simulink model "Simulation"  (R2014b)
settings: Solver=ode3  SolverMode=SingleTasking  StartTime=0.0  StopTime=Sim_time  FixedStep=0.02  RelTol=1e-3
undefined symbols (not defined in the file): A, a, T, thetainit, w, xinit, yinit
settings Model: Creator=Oskar  LastModifiedBy=osklj59
settings OptimizationCC: BlockReduction=off  BooleanDataType=off
settings DebuggingCC: SaveWithParameterizedLinksMsg=none  UnderspecifiedInitializationDetection=Classic  MergeDetectMultiDrivingBlocksExec=none  SignalResolutionControl=TryResolveAllWithWarning  SolverPrmCheckMsg=none
settings HardwareCC: TargetUnknown=on

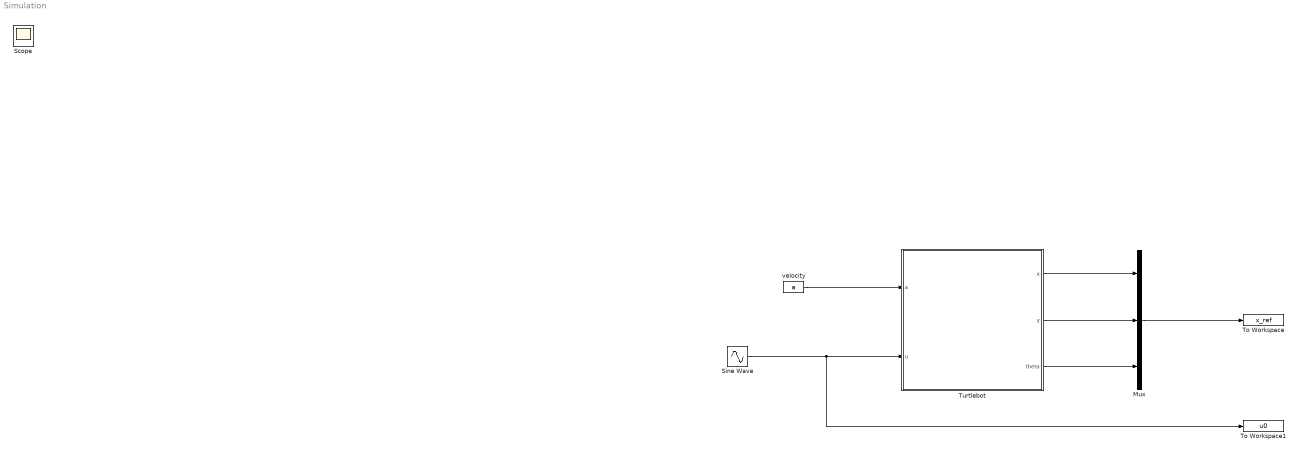
== system Simulation ==
  Mux : Mux  Inputs=3
  Sine Wave : Sin  Amplitude=A  Frequency=w  SampleTime=0
  To Workspace : ToWorkspace  VariableName=x_ref  SaveFormat=Timeseries  SampleTime=-1
  To Workspace1 : ToWorkspace  VariableName=u0  SaveFormat=Timeseries  SampleTime=-1
  Turtlebot : Subsystem
  velocity : Constant  Value=a
  Scope : Scope
      settings: YMin=-0.4  YMax=0.8
  wires:
  Turtlebot/1("x ") -> Mux/1
  Mux/1 -> To Workspace/1
  velocity/1 -> Turtlebot/1(a)
  Turtlebot/2("y ") -> Mux/2
  Turtlebot/3("theta ") -> Mux/3
  Sine Wave/1 -> Turtlebot/2(u), To Workspace1/1

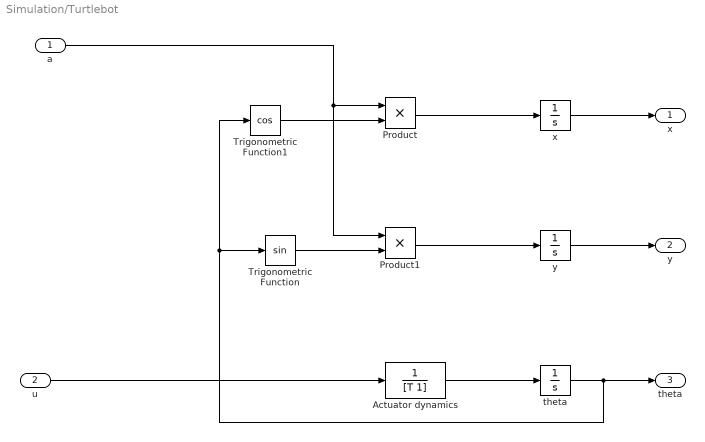
== system Simulation/Turtlebot ==
  a : Inport
  u : Inport  Port=2
  Actuator dynamics : TransferFcn  Denominator=[T 1]
  Product : Product
  Product1 : Product
  Trigonometric Function : Trigonometry
  Trigonometric Function1 : Trigonometry  Operator=cos
  theta : Integrator  InitialCondition=thetainit
  x : Integrator  InitialCondition=xinit
  y : Integrator  InitialCondition=yinit
  "x " : Outport  PortDimensions=1
  "y " : Outport  Port=2
  "theta " : Outport  Port=3
  wires:
  a/1 -> Product1/1, Product/1
  x/1 -> "x "/1
  y/1 -> "y "/1
  theta/1 -> Trigonometric Function1/1, Trigonometric Function/1, "theta "/1
  u/1 -> Actuator dynamics/1
  Trigonometric Function1/1 -> Product/2
  Trigonometric Function/1 -> Product1/2
  Product/1 -> x/1
  Product1/1 -> y/1
  Actuator dynamics/1 -> theta/1
